simulink subsystem "TCS"  (R2025b)
settings: Solver=VariableStepAuto  StartTime=0.0  StopTime=10.0  RelTol=1e-3
libraries: simulink x1, slpidlib x1
settings Model: Creator=mjmag  LastModifiedBy=DIEGO
settings RTWCC: GPUComputeCapability=3.5

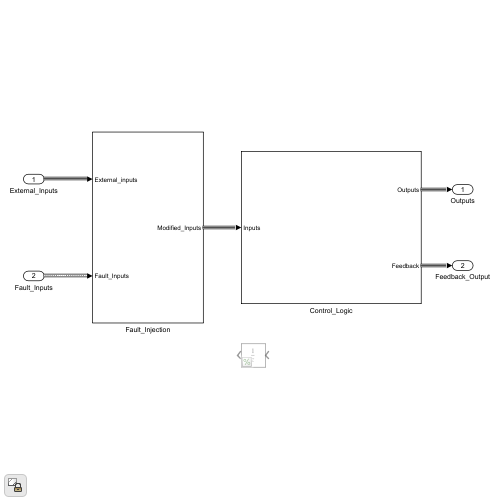
[thumbnail: Simulink's stored preview of the top-level diagram]
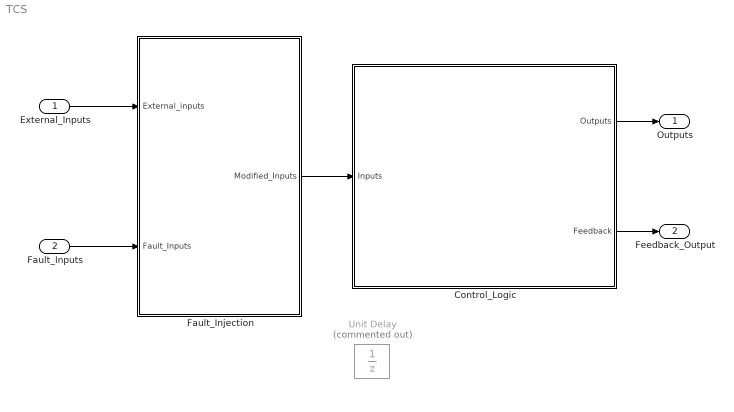
== system TCS ==
  External_Inputs : Inport
  Fault_Inputs : Inport  Port=2
  Control_Logic : Subsystem
  Fault_Injection : Subsystem
  Unit Delay : UnitDelay  Commented=on  SampleTime=-1  HasFrameUpgradeWarning=on
  Outputs : Outport
  Feedback_Output : Outport  Port=2
  wires:
  External_Inputs/1 -> Fault_Injection/1(External_inputs)
  Fault_Inputs/1 -> Fault_Injection/2(Fault_Inputs)
  Control_Logic/2(Feedback) -> Feedback_Output/1
  Control_Logic/1(Outputs) -> Outputs/1
  Fault_Injection/1(Modified_Inputs) -> Control_Logic/1(Inputs)

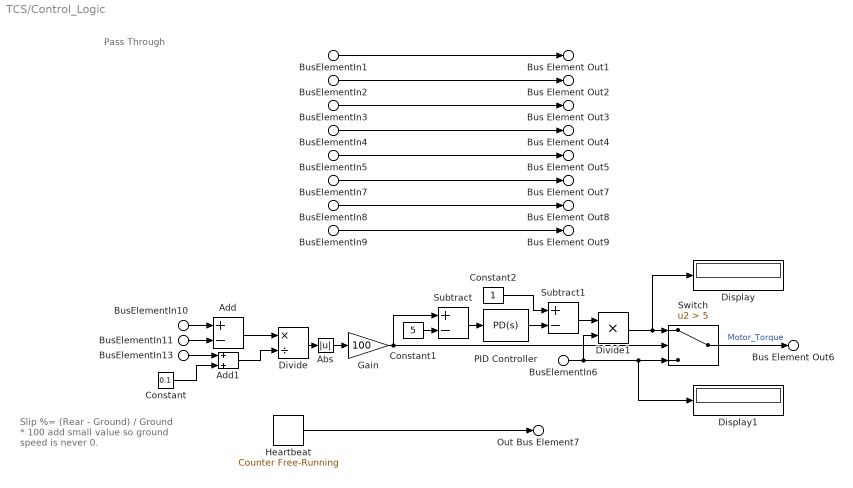
== system TCS/Control_Logic ==
  note: Slip %= (Rear - Ground) / Ground * 100
      | add small value so ground speed is never 0.
  note: Pass Through
  BusElementIn1 : Inport  PortName=Inputs  Element=MC_Outputs
  BusElementIn2 : Inport  PortName=Inputs  Element=LVSS_Outputs
  BusElementIn3 : Inport  PortName=Inputs  Element=TMS_Outputs
  BusElementIn4 : Inport  PortName=Inputs  Element=VCU_Outputs.Inverter_Discharge
  BusElementIn5 : Inport  PortName=Inputs  Element=VCU_Outputs.BMS_Contactor_Command
  BusElementIn6 : Inport  PortName=Inputs  Element=VCU_Outputs.Torque_Command
  BusElementIn7 : Inport  PortName=Inputs  Element=VCU_Outputs.Fault_To_MC
  BusElementIn8 : Inport  PortName=Inputs  Element=VCU_Outputs.Inverter_Enable
  BusElementIn9 : Inport  PortName=Inputs  Element=VCU_Outputs.Shutdown
  BusElementIn10 : Inport  PortName=Inputs  Element=Front_Wheel_Speed
  BusElementIn11 : Inport  PortName=Inputs  Element=Rear_Wheel_Speed
  BusElementIn13 : Inport  PortName=Inputs  Element=Rear_Wheel_Speed
  Abs : Abs  SaturateOnIntegerOverflow=off
  Add : Sum  Inputs=+-
  Add1 : Sum
  Constant : Constant  Value=0.1
  Constant1 : Constant  Value=5
  Constant2 : Constant
  Display : Display
  Display1 : Display
  Divide : Product  Inputs=*/
  Divide1 : Product  Inputs=**
  Gain : Gain  Gain=100
  Heartbeat : simulink/Sources/Counter Free-Running  NumBits=32  tsamp=-1
  PID Controller : slpidlib/PID Controller  Controller=PD  Form=Parallel  TimeDomain=Continuous-time  UseExternalTs=off  SampleTime=-1  IntegratorMethod=Forward Euler  FilterMethod=Forward Euler  ControllerParametersSource=internal  P=0.02  I=5  UseKiTs=off  D=0.01  UseExternalDerivativeSource=off  N=100  UseFilter=on  TunerSelectOption=Transfer Function Based (PID Tuner App)  InitialConditionSource=internal  InitialConditionForIntegrator=0  InitialConditionForFilter=0  DifferentiatorICPrevScaledInput=0  ExternalReset=none  TrackingMode=off  Kt=1  LimitOutput=on  SatLimitsSource=internal  UpperSaturationLimit=0.5  LowerSaturationLimit=0  LinearizeAsGain=on  AntiWindupMode=none  Kb=1  LimitIntegrator=off  UpperIntegratorSaturationLimit=inf  LowerIntegratorSaturationLimit=-inf  POutMin=[]  POutMax=[]  IOutMin=[]  IOutMax=[]  DOutMin=[]  DOutMax=[]  NOutMin=[]  NOutMax=[]  SumOutMin=[]  SumOutMax=[]  SaturationOutMin=[]  SaturationOutMax=[]  PParamMin=[]  PParamMax=[]  IParamMin=[]  IParamMax=[]  DParamMin=[]  DParamMax=[]  NParamMin=[]  NParamMax=[]  KbParamMin=[]  KbParamMax=[]  KtParamMin=[]  KtParamMax=[]  KbOutMin=[]  KbOutMax=[]  KtOutMin=[]  KtOutMax=[]  IntegratorOutMin=[]  IntegratorOutMax=[]  FilterOutMin=[]  FilterOutMax=[]  SumI1OutMin=[]  SumI1OutMax=[]  SumI2OutMin=[]  SumI2OutMax=[]  SumI3OutMin=[]  SumI3OutMax=[]  SumI4OutMin=[]  SumI4OutMax=[]  SumDOutMin=[]  SumDOutMax=[]  DifferentiatorOutMin=[]  DifferentiatorOutMax=[]  FilterDiffOutCoefMin=[]  FilterDiffOutCoefMax=[]  ReciprocalOutMin=[]  ReciprocalOutMax=[]  SumDenOutMin=[]  SumDenOutMax=[]  SumNumOutMin=[]  SumNumOutMax=[]  DivideOutMin=[]  DivideOutMax=[]  UdiffTsProdOutMin=[]  UdiffTsProdOutMax=[]  NTsProdOutMin=[]  NTsProdOutMax=[]  UintegralTsProdOutMin=[]  UintegralTsProdOutMax=[]  UngainTsProdOutMin=[]  UngainTsProdOutMax=[]  ClampingZeroOutDataTypeStr=Inherit: Inherit via back propagation  ClampingZeroOutMin=[]  ClampingZeroOutMax=[]  FilterDenConstantOutDataTypeStr=Inherit: Inherit via back propagation  FilterDenConstantOutMin=[]  FilterDenConstantOutMax=[]  PCopyOutDataTypeStr=Inherit: Inherit via back propagation  PCopyOutMin=[]  PCopyOutMax=[]  NCopyOutDataTypeStr=Inherit: Inherit via back propagation  NCopyOutMin=[]  NCopyOutMax=[]  IntegratorContinuousStateAttributes=''  IntegratorStateMustResolveToSignalObject=off  IntegratorRTWStateStorageClass=Auto  FilterContinuousStateAttributes=''  FilterStateMustResolveToSignalObject=off  FilterRTWStateStorageClass=Auto  ParallelPVariant=InternalParameters  IdealPVariant=Disabled  IVariant=Disabled  DVariant=InternalParameters  IntegratorVariant=Disabled  SatVariant=Enabled  AWVariant=Disabled  PCopyVariant=Disabled  TRVariant=Disabled  FdbkBlocksVariant=Forward  IdealPFdbkVariant=Disabled  SatFdbkVariant=Disabled  DerivativeFilterVariant=ContFilter  NVariant=InternalParameters  NCopyVariant=Disabled  FilterICVariant=InternalICsFilter  IntegratorICVariant=Disabled  ExternalResetVariant=Disabled  TRSumVariant=Passthrough  SumFdbkVariant=Disabled  SumVariant=Sum_PD  TsampFilterVariant=InternalTs  TsampNgainVariant=Passthrough  TsampIntegralVariant=Disabled_SignalSpec  ExternalSaturationOutDataTypeStr=Inherit: Same as second input  DerivativeSourceVariant=ErrorSignal  PreIntVariant=InternalPreInt
  Subtract : Sum  Inputs=+-
  Subtract1 : Sum  Inputs=+-
  Switch : Switch  Criteria=u2 > Threshold  Threshold=5  SaturateOnIntegerOverflow=off  InputSameDT=off
  Bus Element Out1 : Outport  PortName=Outputs  Element=MC_Outputs
  Bus Element Out2 : Outport  PortName=Outputs  Element=LVSS_Outputs
  Bus Element Out3 : Outport  PortName=Outputs  Element=TMS_Outputs
  Bus Element Out4 : Outport  PortName=Outputs  Element=VCU_Outputs.Inverter_Discharge
  Bus Element Out5 : Outport  PortName=Outputs  Element=VCU_Outputs.BMS_Contactor_Command
  Bus Element Out6 : Outport  PortName=Outputs  Element=VCU_Outputs.Torque_Command
  Bus Element Out7 : Outport  PortName=Outputs  Element=VCU_Outputs.Fault_To_MC
  Bus Element Out8 : Outport  PortName=Outputs  Element=VCU_Outputs.Inverter_Enable
  Bus Element Out9 : Outport  PortName=Outputs  Element=VCU_Outputs.Shutdown
  Out Bus Element7 : Outport  Port=2  PortName=Feedback  Element=TCS_Heartbeat
  wires:
  Abs/1 -> Gain/1
  Divide/1 -> Abs/1
  Constant/1 -> Add1/2
  Add1/1 -> Divide/2
  Switch/1 -> Bus Element Out6/1  "Motor_Torque"
  BusElementIn6/1 -> Switch/3, Display1/1, Divide1/2
  Constant2/1 -> Subtract1/1
  Subtract1/1 -> Divide1/1
  Constant1/1 -> Subtract/2
  Add/1 -> Divide/1
  Subtract/1 -> PID Controller/1
  Divide1/1 -> Switch/1, Display/1
  PID Controller/1 -> Subtract1/2
  Gain/1 -> Switch/2, Subtract/1
  BusElementIn13/1 -> Add1/1
  BusElementIn11/1 -> Add/2
  BusElementIn10/1 -> Add/1
  BusElementIn9/1 -> Bus Element Out9/1
  BusElementIn8/1 -> Bus Element Out8/1
  BusElementIn7/1 -> Bus Element Out7/1
  BusElementIn5/1 -> Bus Element Out5/1
  BusElementIn4/1 -> Bus Element Out4/1
  BusElementIn3/1 -> Bus Element Out3/1
  BusElementIn2/1 -> Bus Element Out2/1
  Heartbeat/1 -> Out Bus Element7/1
  BusElementIn1/1 -> Bus Element Out1/1

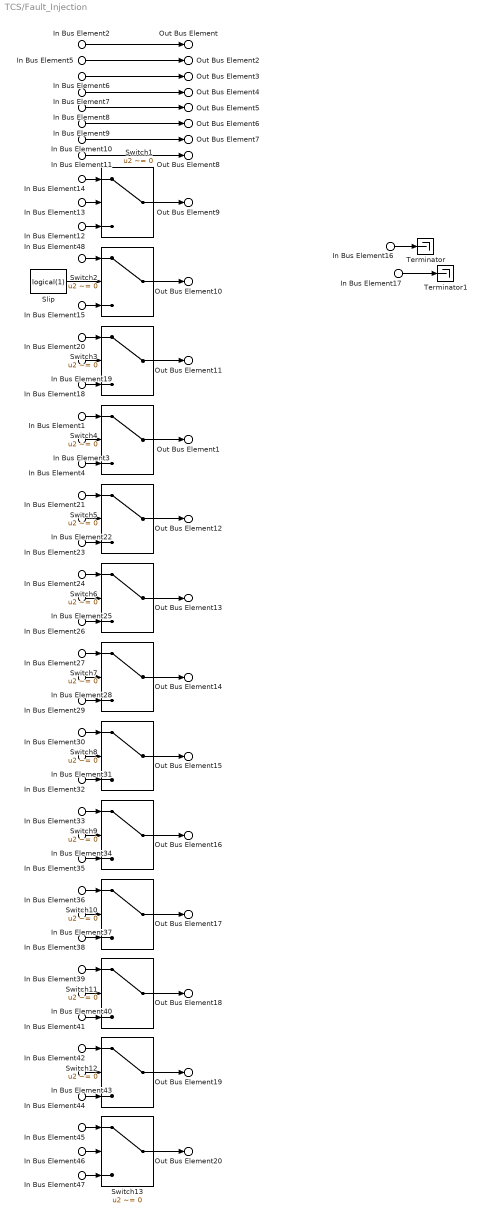
== system TCS/Fault_Injection ==
  In Bus Element2 : Inport  PortName=External_inputs  Element=VCU.MC_Outputs
  In Bus Element5 : Inport  PortName=External_inputs  Element=VCU.LVSS_Outputs
  In Bus Element6 : Inport  PortName=External_inputs  Element=VCU.TMS_Outputs
  In Bus Element7 : Inport  PortName=External_inputs  Element=VCU.VCU_Outputs.Inverter_Discharge
  In Bus Element8 : Inport  PortName=External_inputs  Element=VCU.VCU_Outputs.BMS_Contactor_Command
  In Bus Element9 : Inport  PortName=External_inputs  Element=VCU.VCU_Outputs.Fault_To_MC
  In Bus Element10 : Inport  PortName=External_inputs  Element=VCU.VCU_Outputs.Inverter_Enable
  In Bus Element11 : Inport  PortName=External_inputs  Element=VCU.VCU_Outputs.Shutdown
  In Bus Element12 : Inport  PortName=External_inputs  Element=VCU.VCU_Outputs.Torque_Command
  In Bus Element15 : Inport  PortName=External_inputs  Element=WSS.WSS_Front_Wheel_Speed
  In Bus Element18 : Inport  PortName=External_inputs  Element=WSS.WSS_Rear_Wheel_Speed
  In Bus Element4 : Inport  PortName=External_inputs  Element=INS.Acceleration_X
  In Bus Element23 : Inport  PortName=External_inputs  Element=INS.Acceleration_Y
  In Bus Element26 : Inport  PortName=External_inputs  Element=INS.Acceleration_Z
  In Bus Element29 : Inport  PortName=External_inputs  Element=INS.Ground_Speed
  In Bus Element32 : Inport  PortName=External_inputs  Element=INS.Yaw
  In Bus Element35 : Inport  PortName=External_inputs  Element=INS.Pitch
  In Bus Element38 : Inport  PortName=External_inputs  Element=INS.Roll
  In Bus Element41 : Inport  PortName=External_inputs  Element=INS.Roll_Rate
  In Bus Element44 : Inport  PortName=External_inputs  Element=INS.Pitch_Rate
  In Bus Element47 : Inport  PortName=External_inputs  Element=INS.Yaw_Rate
  In Bus Element48 : Inport  PortName=External_inputs  Element=WSS_Fake.WSS_Wheel_Speed
  In Bus Element14 : Inport  Port=2  PortName=Fault_Inputs  Element=VCU_Torque_Command
  In Bus Element13 : Inport  Port=2  PortName=Fault_Inputs  Element=Override_VCU_Torque_Command
  In Bus Element16 : Inport  Port=2  PortName=Fault_Inputs  Element=Front_Wheel_Speed
  In Bus Element17 : Inport  Port=2  PortName=Fault_Inputs  Element=Override_Front_Wheel_Speed
  In Bus Element19 : Inport  Port=2  PortName=Fault_Inputs  Element=Override_Rear_Wheel_Speed
  In Bus Element20 : Inport  Port=2  PortName=Fault_Inputs  Element=Rear_Wheel_Speed
  In Bus Element1 : Inport  Port=2  PortName=Fault_Inputs  Element=Acceleration_X
  In Bus Element3 : Inport  Port=2  PortName=Fault_Inputs  Element=Override_Acceleration_X
  In Bus Element21 : Inport  Port=2  PortName=Fault_Inputs  Element=Acceleration_Y
  In Bus Element22 : Inport  Port=2  PortName=Fault_Inputs  Element=Override_Acceleration_Y
  In Bus Element24 : Inport  Port=2  PortName=Fault_Inputs  Element=Acceleration_Z
  In Bus Element25 : Inport  Port=2  PortName=Fault_Inputs  Element=Override_Acceleration_Z
  In Bus Element27 : Inport  Port=2  PortName=Fault_Inputs  Element=Ground_Speed
  In Bus Element28 : Inport  Port=2  PortName=Fault_Inputs  Element=Override_Ground_Speed
  In Bus Element30 : Inport  Port=2  PortName=Fault_Inputs  Element=Yaw
  In Bus Element31 : Inport  Port=2  PortName=Fault_Inputs  Element=Override_Yaw
  In Bus Element33 : Inport  Port=2  PortName=Fault_Inputs  Element=Pitch
  In Bus Element34 : Inport  Port=2  PortName=Fault_Inputs  Element=Override_Pitch
  In Bus Element36 : Inport  Port=2  PortName=Fault_Inputs  Element=Roll
  In Bus Element37 : Inport  Port=2  PortName=Fault_Inputs  Element=Override_Roll
  In Bus Element39 : Inport  Port=2  PortName=Fault_Inputs  Element=Roll_Rate
  In Bus Element40 : Inport  Port=2  PortName=Fault_Inputs  Element=Override_Roll_Rate
  In Bus Element42 : Inport  Port=2  PortName=Fault_Inputs  Element=Pitch_Rate
  In Bus Element43 : Inport  Port=2  PortName=Fault_Inputs  Element=Override_Pitch_Rate
  In Bus Element45 : Inport  Port=2  PortName=Fault_Inputs  Element=Yaw_Rate
  In Bus Element46 : Inport  Port=2  PortName=Fault_Inputs  Element=Override_Yaw_Rate
  Slip : Constant  Value=logical(1)
  Switch{1..13} (13 alike) : Switch  Criteria=u2 ~= 0  SaturateOnIntegerOverflow=off  InputSameDT=off
  Terminator : Terminator
  Terminator1 : Terminator
  Out Bus Element : Outport  PortName=Modified_Inputs  Element=MC_Outputs
  Out Bus Element2 : Outport  PortName=Modified_Inputs  Element=LVSS_Outputs
  Out Bus Element3 : Outport  PortName=Modified_Inputs  Element=TMS_Outputs
  Out Bus Element4 : Outport  PortName=Modified_Inputs  Element=VCU_Outputs.Inverter_Discharge
  Out Bus Element5 : Outport  PortName=Modified_Inputs  Element=VCU_Outputs.BMS_Contactor_Command
  Out Bus Element6 : Outport  PortName=Modified_Inputs  Element=VCU_Outputs.Fault_To_MC
  Out Bus Element7 : Outport  PortName=Modified_Inputs  Element=VCU_Outputs.Inverter_Enable
  Out Bus Element8 : Outport  PortName=Modified_Inputs  Element=VCU_Outputs.Shutdown
  Out Bus Element9 : Outport  PortName=Modified_Inputs  Element=VCU_Outputs.Torque_Command
  Out Bus Element10 : Outport  PortName=Modified_Inputs  Element=Front_Wheel_Speed
  Out Bus Element11 : Outport  PortName=Modified_Inputs  Element=Rear_Wheel_Speed
  Out Bus Element1 : Outport  PortName=Modified_Inputs  Element=Acceleration_X
  Out Bus Element12 : Outport  PortName=Modified_Inputs  Element=Acceleration_Y
  Out Bus Element13 : Outport  PortName=Modified_Inputs  Element=Acceleration_Z
  Out Bus Element14 : Outport  PortName=Modified_Inputs  Element=Ground_Speed
  Out Bus Element15 : Outport  PortName=Modified_Inputs  Element=Yaw
  Out Bus Element16 : Outport  PortName=Modified_Inputs  Element=Pitch
  Out Bus Element17 : Outport  PortName=Modified_Inputs  Element=Roll
  Out Bus Element18 : Outport  PortName=Modified_Inputs  Element=Roll_Rate
  Out Bus Element19 : Outport  PortName=Modified_Inputs  Element=Pitch_Rate
  Out Bus Element20 : Outport  PortName=Modified_Inputs  Element=Yaw_Rate
  wires:
  Slip/1 -> Switch2/2
  In Bus Element48/1 -> Switch2/1
  Switch13/1 -> Out Bus Element20/1
  In Bus Element47/1 -> Switch13/3
  In Bus Element46/1 -> Switch13/2
  In Bus Element45/1 -> Switch13/1
  In Bus Element44/1 -> Switch12/3
  In Bus Element43/1 -> Switch12/2
  In Bus Element42/1 -> Switch12/1
  Switch12/1 -> Out Bus Element19/1
  Switch11/1 -> Out Bus Element18/1
  In Bus Element41/1 -> Switch11/3
  In Bus Element40/1 -> Switch11/2
  In Bus Element39/1 -> Switch11/1
  Switch10/1 -> Out Bus Element17/1
  In Bus Element38/1 -> Switch10/3
  In Bus Element37/1 -> Switch10/2
  In Bus Element36/1 -> Switch10/1
  Switch9/1 -> Out Bus Element16/1
  In Bus Element35/1 -> Switch9/3
  In Bus Element34/1 -> Switch9/2
  In Bus Element33/1 -> Switch9/1
  Switch8/1 -> Out Bus Element15/1
  In Bus Element32/1 -> Switch8/3
  In Bus Element31/1 -> Switch8/2
  In Bus Element30/1 -> Switch8/1
  Switch7/1 -> Out Bus Element14/1
  In Bus Element29/1 -> Switch7/3
  In Bus Element28/1 -> Switch7/2
  In Bus Element27/1 -> Switch7/1
  Switch6/1 -> Out Bus Element13/1
  In Bus Element26/1 -> Switch6/3
  In Bus Element25/1 -> Switch6/2
  In Bus Element24/1 -> Switch6/1
  Switch5/1 -> Out Bus Element12/1
  In Bus Element23/1 -> Switch5/3
  In Bus Element22/1 -> Switch5/2
  In Bus Element21/1 -> Switch5/1
  Switch4/1 -> Out Bus Element1/1
  In Bus Element4/1 -> Switch4/3
  In Bus Element3/1 -> Switch4/2
  In Bus Element1/1 -> Switch4/1
  Switch3/1 -> Out Bus Element11/1
  In Bus Element18/1 -> Switch3/3
  In Bus Element19/1 -> Switch3/2
  In Bus Element20/1 -> Switch3/1
  Switch2/1 -> Out Bus Element10/1
  In Bus Element16/1 -> Terminator/1
  In Bus Element15/1 -> Switch2/3
  In Bus Element17/1 -> Terminator1/1
  Switch1/1 -> Out Bus Element9/1
  In Bus Element14/1 -> Switch1/1
  In Bus Element12/1 -> Switch1/3
  In Bus Element13/1 -> Switch1/2
  In Bus Element11/1 -> Out Bus Element8/1
  In Bus Element10/1 -> Out Bus Element7/1
  In Bus Element9/1 -> Out Bus Element6/1
  In Bus Element8/1 -> Out Bus Element5/1
  In Bus Element7/1 -> Out Bus Element4/1
  In Bus Element6/1 -> Out Bus Element3/1
  In Bus Element5/1 -> Out Bus Element2/1
  In Bus Element2/1 -> Out Bus Element/1
